simulink model "NO3_Multi_QuadcopterOffboard_Actuator"  (R2022a)
settings: Solver=FixedStepAuto  StartTime=0.0  StopTime=inf  RelTol=1e-3
undefined symbols (not defined in the file): actuator, command, control, param1, param2, target_system, timestamp
libraries: ros2lib x33
settings Model: Creator=liuwhale  LastModifiedBy=liuwhale
settings OptimizationCC: EnhancedBackFolding=on  PassReuseOutputArgsAs=Individual arguments  ZeroExternalMemoryAtStartup=off  ZeroInternalMemoryAtStartup=off  MaxStackSize=64  OptimizeBlockOrder=speed  DifferentSizesBufferReuse=on  OptimizationCustomize=off  EfficientTunableParamExpr=on
settings DebuggingCC: ParameterTunabilityLossMsg=error
settings SFSimCC: MATLABDynamicMemAlloc=off
settings RTWCC: SystemTargetFile=ert.tlc  HardwareBoard=Robot Operating System 2 (ROS 2)  TLCOptions="-aInlineSetEventsForThisBaseRateFcn=TLC_FALSE -aSuppressMultiTaskScheduler=TLC_FALSE  -aRateBasedStepFcn=0"  TemplateMakefile=ert_default_tmf  Toolchain=Colcon Tools  TargetLang=C++
settings CodeAppCC: ForceParamTrailComments=on  IgnoreCustomStorageClasses=off  OperatorAnnotations=on  SimulinkDataObjDesc=on  SFDataObjDesc=on  InsertBlockDesc=on
settings ERTTargetCC: CodeInterfacePackaging=C++ class  RootIOFormat=Structure reference

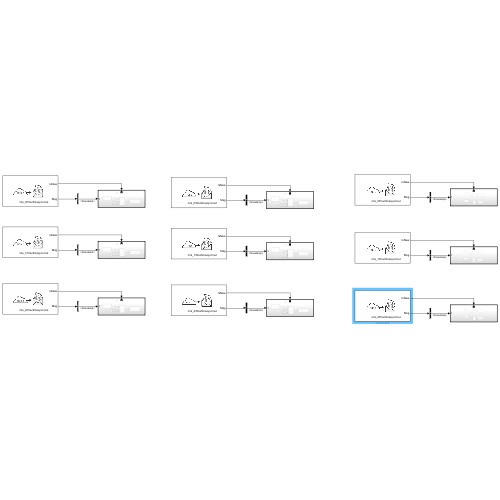
[thumbnail: Simulink's stored preview of the top-level diagram]
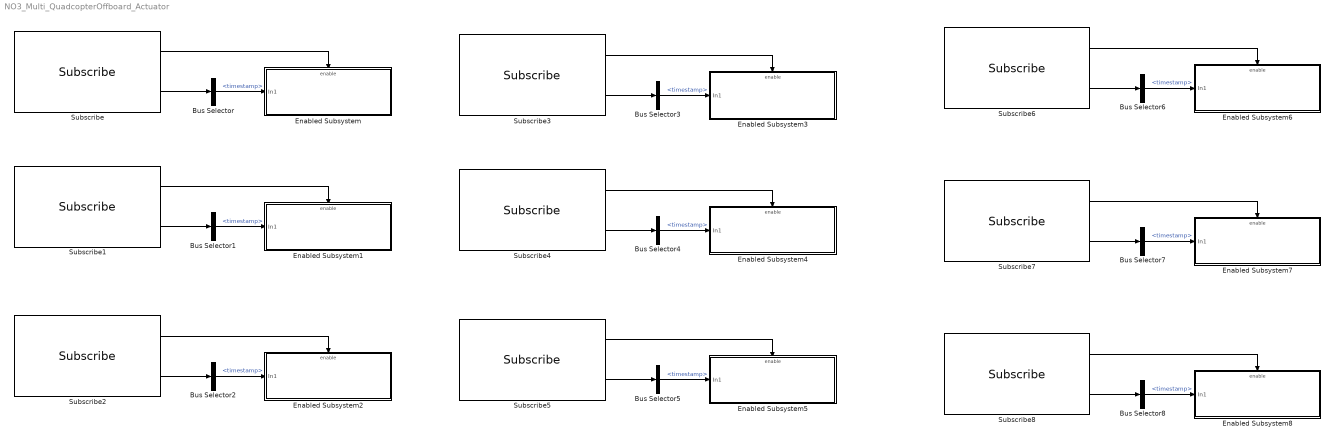
== system NO3_Multi_QuadcopterOffboard_Actuator ==
  Bus Selector{,1..8} (9 alike) : BusSelector  OutputSignals=timestamp
  Enabled Subsystem : Subsystem  TreatAsAtomicUnit=on
  Enabled Subsystem1 : Subsystem  TreatAsAtomicUnit=on
  Enabled Subsystem2 : Subsystem  TreatAsAtomicUnit=on
  Enabled Subsystem3 : Subsystem  TreatAsAtomicUnit=on
  Enabled Subsystem4 : Subsystem  TreatAsAtomicUnit=on
  Enabled Subsystem5 : Subsystem  TreatAsAtomicUnit=on
  Enabled Subsystem6 : Subsystem  TreatAsAtomicUnit=on
  Enabled Subsystem7 : Subsystem  TreatAsAtomicUnit=on
  Enabled Subsystem8 : Subsystem  TreatAsAtomicUnit=on
  Subscribe : ros2lib/Subscribe  topicSource=Specify your own  topic=/iris_0/fmu/timesync/out  messageType=px4_msgs/Timesync  sampleTime=-1  QOSHistory=Keep last  QOSDepth=1  QOSReliability=Reliable  QOSDurability=Volatile
      settings: SourceProductBaseCode=RR
  Subscribe1 : ros2lib/Subscribe  topicSource=Specify your own  topic=/iris_1/fmu/timesync/out  messageType=px4_msgs/Timesync  sampleTime=-1  QOSHistory=Keep last  QOSDepth=1  QOSReliability=Reliable  QOSDurability=Volatile
      settings: SourceProductBaseCode=RR
  Subscribe2 : ros2lib/Subscribe  topicSource=Specify your own  topic=/iris_2/fmu/timesync/out  messageType=px4_msgs/Timesync  sampleTime=-1  QOSHistory=Keep last  QOSDepth=1  QOSReliability=Reliable  QOSDurability=Volatile
      settings: SourceProductBaseCode=RR
  Subscribe3 : ros2lib/Subscribe  topicSource=Specify your own  topic=/iris_0/fmu/timesync/out  messageType=px4_msgs/Timesync  sampleTime=-1  QOSHistory=Keep last  QOSDepth=1  QOSReliability=Reliable  QOSDurability=Volatile
      settings: SourceProductBaseCode=RR
  Subscribe4 : ros2lib/Subscribe  topicSource=Specify your own  topic=/iris_1/fmu/timesync/out  messageType=px4_msgs/Timesync  sampleTime=-1  QOSHistory=Keep last  QOSDepth=1  QOSReliability=Reliable  QOSDurability=Volatile
      settings: SourceProductBaseCode=RR
  Subscribe5 : ros2lib/Subscribe  topicSource=Specify your own  topic=/iris_2/fmu/timesync/out  messageType=px4_msgs/Timesync  sampleTime=-1  QOSHistory=Keep last  QOSDepth=1  QOSReliability=Reliable  QOSDurability=Volatile
      settings: SourceProductBaseCode=RR
  Subscribe6 : ros2lib/Subscribe  topicSource=Specify your own  topic=/iris_0/fmu/timesync/out  messageType=px4_msgs/Timesync  sampleTime=-1  QOSHistory=Keep last  QOSDepth=1  QOSReliability=Reliable  QOSDurability=Volatile
      settings: SourceProductBaseCode=RR
  Subscribe7 : ros2lib/Subscribe  topicSource=Specify your own  topic=/iris_1/fmu/timesync/out  messageType=px4_msgs/Timesync  sampleTime=-1  QOSHistory=Keep last  QOSDepth=1  QOSReliability=Reliable  QOSDurability=Volatile
      settings: SourceProductBaseCode=RR
  Subscribe8 : ros2lib/Subscribe  topicSource=Specify your own  topic=/iris_2/fmu/timesync/out  messageType=px4_msgs/Timesync  sampleTime=-1  QOSHistory=Keep last  QOSDepth=1  QOSReliability=Reliable  QOSDurability=Volatile
      settings: SourceProductBaseCode=RR
  wires:
  Subscribe/1 -> Enabled Subsystem/Enable
  Subscribe/2 -> Bus Selector/1
  Bus Selector/1 -> Enabled Subsystem/1(In1)  "<timestamp>"
  Bus Selector1/1 -> Enabled Subsystem1/1(In1)  "<timestamp>"
  Subscribe1/2 -> Bus Selector1/1
  Subscribe1/1 -> Enabled Subsystem1/Enable
  Bus Selector2/1 -> Enabled Subsystem2/1(In1)  "<timestamp>"
  Subscribe2/2 -> Bus Selector2/1
  Subscribe2/1 -> Enabled Subsystem2/Enable
  Subscribe5/1 -> Enabled Subsystem5/Enable
  Bus Selector5/1 -> Enabled Subsystem5/1(In1)  "<timestamp>"
  Subscribe5/2 -> Bus Selector5/1
  Subscribe4/2 -> Bus Selector4/1
  Subscribe4/1 -> Enabled Subsystem4/Enable
  Bus Selector3/1 -> Enabled Subsystem3/1(In1)  "<timestamp>"
  Subscribe3/2 -> Bus Selector3/1
  Subscribe3/1 -> Enabled Subsystem3/Enable
  Bus Selector4/1 -> Enabled Subsystem4/1(In1)  "<timestamp>"
  Subscribe6/2 -> Bus Selector6/1
  Bus Selector6/1 -> Enabled Subsystem6/1(In1)  "<timestamp>"
  Subscribe6/1 -> Enabled Subsystem6/Enable
  Subscribe7/2 -> Bus Selector7/1
  Bus Selector7/1 -> Enabled Subsystem7/1(In1)  "<timestamp>"
  Subscribe8/2 -> Bus Selector8/1
  Bus Selector8/1 -> Enabled Subsystem8/1(In1)  "<timestamp>"
  Subscribe7/1 -> Enabled Subsystem7/Enable
  Subscribe8/1 -> Enabled Subsystem8/Enable

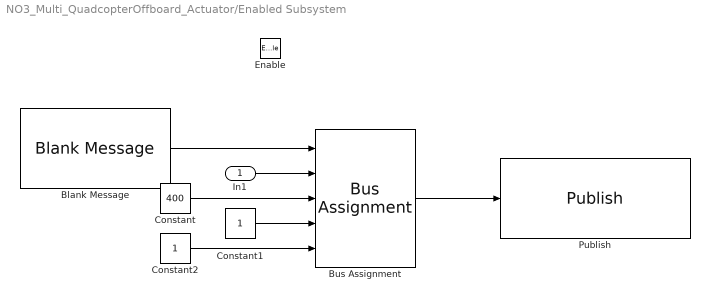
== system NO3_Multi_QuadcopterOffboard_Actuator/Enabled Subsystem ==
  In1 : Inport
  Enable : EnablePort
  Blank Message : ros2lib/Blank Message  messageClass=Message  entityType=px4_msgs/VehicleCommand  messageType=px4_msgs/VehicleCommand  SampleTime=inf
      settings: SourceProductBaseCode=RR
  Bus Assignment : BusAssignment  AssignedSignals=timestamp,command,param1,target_system
  Constant : Constant  Value=400  OutDataTypeStr=uint32
  Constant1 : Constant  OutDataTypeStr=single
  Constant2 : Constant  OutDataTypeStr=uint8
  Publish : ros2lib/Publish  topicSource=Specify your own  topic=/iris_0/fmu/vehicle_command/in  messageType=px4_msgs/VehicleCommand  QOSHistory=Keep last  QOSDepth=1  QOSReliability=Reliable  QOSDurability=Volatile
      settings: SourceProductBaseCode=RR
  wires:
  Blank Message/1 -> Bus Assignment/1
  In1/1 -> Bus Assignment/2
  Constant/1 -> Bus Assignment/3
  Constant1/1 -> Bus Assignment/4
  Constant2/1 -> Bus Assignment/5
  Bus Assignment/1 -> Publish/1

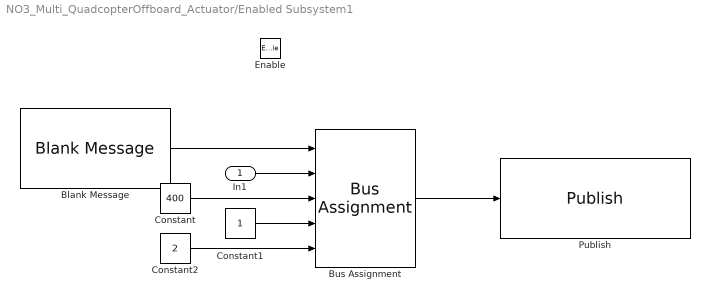
== system NO3_Multi_QuadcopterOffboard_Actuator/Enabled Subsystem1 ==
  In1 : Inport
  Enable : EnablePort
  Blank Message : ros2lib/Blank Message  messageClass=Message  entityType=px4_msgs/VehicleCommand  messageType=px4_msgs/VehicleCommand  SampleTime=inf
      settings: SourceProductBaseCode=RR
  Bus Assignment : BusAssignment  AssignedSignals=timestamp,command,param1,target_system
  Constant : Constant  Value=400  OutDataTypeStr=uint32
  Constant1 : Constant  OutDataTypeStr=single
  Constant2 : Constant  Value=2  OutDataTypeStr=uint8
  Publish : ros2lib/Publish  topicSource=Specify your own  topic=/iris_1/fmu/vehicle_command/in  messageType=px4_msgs/VehicleCommand  QOSHistory=Keep last  QOSDepth=1  QOSReliability=Reliable  QOSDurability=Volatile
      settings: SourceProductBaseCode=RR
  wires:
  Blank Message/1 -> Bus Assignment/1
  In1/1 -> Bus Assignment/2
  Constant/1 -> Bus Assignment/3
  Constant1/1 -> Bus Assignment/4
  Constant2/1 -> Bus Assignment/5
  Bus Assignment/1 -> Publish/1

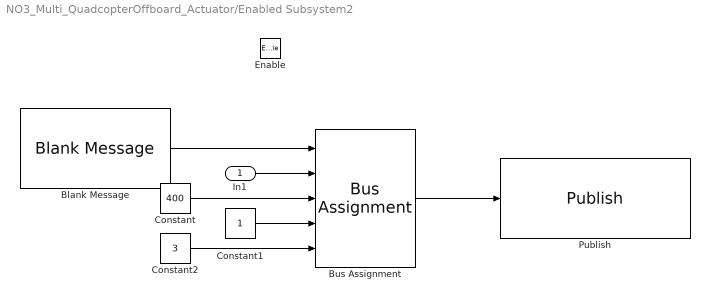
== system NO3_Multi_QuadcopterOffboard_Actuator/Enabled Subsystem2 ==
  In1 : Inport
  Enable : EnablePort
  Blank Message : ros2lib/Blank Message  messageClass=Message  entityType=px4_msgs/VehicleCommand  messageType=px4_msgs/VehicleCommand  SampleTime=inf
      settings: SourceProductBaseCode=RR
  Bus Assignment : BusAssignment  AssignedSignals=timestamp,command,param1,target_system
  Constant : Constant  Value=400  OutDataTypeStr=uint32
  Constant1 : Constant  OutDataTypeStr=single
  Constant2 : Constant  Value=3  OutDataTypeStr=uint8
  Publish : ros2lib/Publish  topicSource=Specify your own  topic=/iris_2/fmu/vehicle_command/in  messageType=px4_msgs/VehicleCommand  QOSHistory=Keep last  QOSDepth=1  QOSReliability=Reliable  QOSDurability=Volatile
      settings: SourceProductBaseCode=RR
  wires:
  Blank Message/1 -> Bus Assignment/1
  In1/1 -> Bus Assignment/2
  Constant/1 -> Bus Assignment/3
  Constant1/1 -> Bus Assignment/4
  Constant2/1 -> Bus Assignment/5
  Bus Assignment/1 -> Publish/1

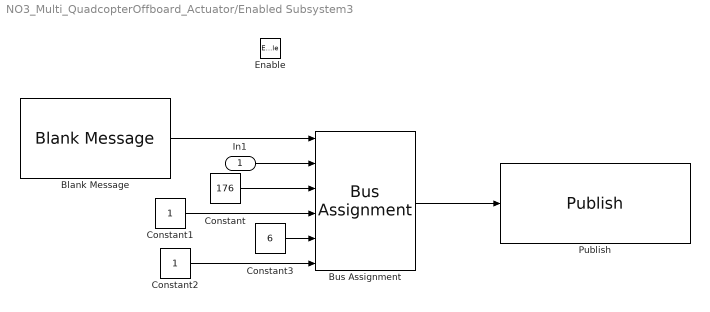
== system NO3_Multi_QuadcopterOffboard_Actuator/Enabled Subsystem3 ==
  In1 : Inport
  Enable : EnablePort
  Blank Message : ros2lib/Blank Message  messageClass=Message  entityType=px4_msgs/VehicleCommand  messageType=px4_msgs/VehicleCommand  SampleTime=inf
      settings: SourceProductBaseCode=RR
  Bus Assignment : BusAssignment  AssignedSignals=timestamp,command,param1,param2,target_system
  Constant : Constant  Value=176  OutDataTypeStr=uint32
  Constant1 : Constant  OutDataTypeStr=single
  Constant2 : Constant  OutDataTypeStr=uint8
  Constant3 : Constant  Value=6  OutDataTypeStr=single
  Publish : ros2lib/Publish  topicSource=Specify your own  topic=/iris_0/fmu/vehicle_command/in  messageType=px4_msgs/VehicleCommand  QOSHistory=Keep last  QOSDepth=1  QOSReliability=Reliable  QOSDurability=Volatile
      settings: SourceProductBaseCode=RR
  wires:
  Blank Message/1 -> Bus Assignment/1
  In1/1 -> Bus Assignment/2
  Constant/1 -> Bus Assignment/3
  Constant1/1 -> Bus Assignment/4
  Constant2/1 -> Bus Assignment/6
  Bus Assignment/1 -> Publish/1
  Constant3/1 -> Bus Assignment/5

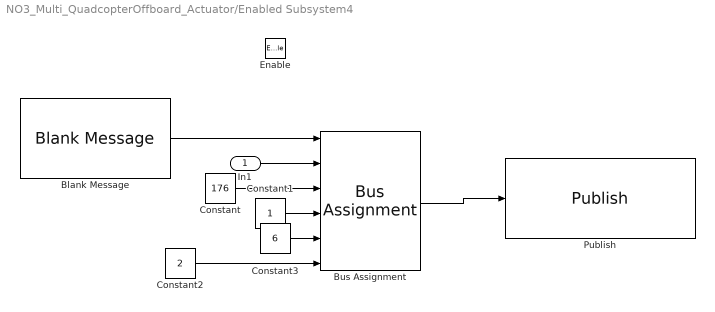
== system NO3_Multi_QuadcopterOffboard_Actuator/Enabled Subsystem4 ==
  In1 : Inport
  Enable : EnablePort
  Blank Message : ros2lib/Blank Message  messageClass=Message  entityType=px4_msgs/VehicleCommand  messageType=px4_msgs/VehicleCommand  SampleTime=inf
      settings: SourceProductBaseCode=RR
  Bus Assignment : BusAssignment  AssignedSignals=timestamp,command,param1,param2,target_system
  Constant : Constant  Value=176  OutDataTypeStr=uint32
  Constant1 : Constant  OutDataTypeStr=single
  Constant2 : Constant  Value=2  OutDataTypeStr=uint8
  Constant3 : Constant  Value=6  OutDataTypeStr=single
  Publish : ros2lib/Publish  topicSource=Specify your own  topic=/iris_1/fmu/vehicle_command/in  messageType=px4_msgs/VehicleCommand  QOSHistory=Keep last  QOSDepth=1  QOSReliability=Reliable  QOSDurability=Volatile
      settings: SourceProductBaseCode=RR
  wires:
  Blank Message/1 -> Bus Assignment/1
  In1/1 -> Bus Assignment/2
  Constant/1 -> Bus Assignment/3
  Constant1/1 -> Bus Assignment/4
  Constant2/1 -> Bus Assignment/6
  Bus Assignment/1 -> Publish/1
  Constant3/1 -> Bus Assignment/5

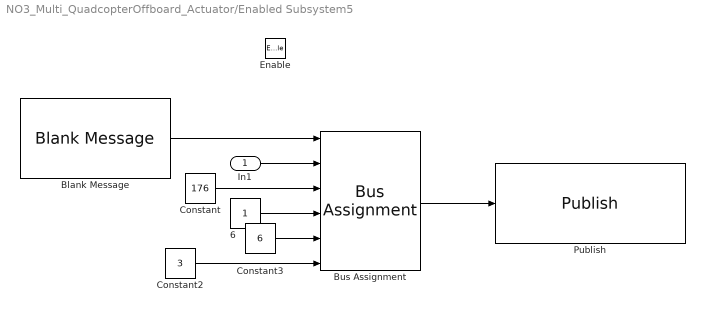
== system NO3_Multi_QuadcopterOffboard_Actuator/Enabled Subsystem5 ==
  In1 : Inport
  Enable : EnablePort
  6 : Constant  OutDataTypeStr=single
  Blank Message : ros2lib/Blank Message  messageClass=Message  entityType=px4_msgs/VehicleCommand  messageType=px4_msgs/VehicleCommand  SampleTime=inf
      settings: SourceProductBaseCode=RR
  Bus Assignment : BusAssignment  AssignedSignals=timestamp,command,param1,param2,target_system
  Constant : Constant  Value=176  OutDataTypeStr=uint32
  Constant2 : Constant  Value=3  OutDataTypeStr=uint8
  Constant3 : Constant  Value=6  OutDataTypeStr=single
  Publish : ros2lib/Publish  topicSource=Specify your own  topic=/iris_2/fmu/vehicle_command/in  messageType=px4_msgs/VehicleCommand  QOSHistory=Keep last  QOSDepth=1  QOSReliability=Reliable  QOSDurability=Volatile
      settings: SourceProductBaseCode=RR
  wires:
  Blank Message/1 -> Bus Assignment/1
  In1/1 -> Bus Assignment/2
  Constant/1 -> Bus Assignment/3
  6/1 -> Bus Assignment/4
  Constant2/1 -> Bus Assignment/6
  Bus Assignment/1 -> Publish/1
  Constant3/1 -> Bus Assignment/5

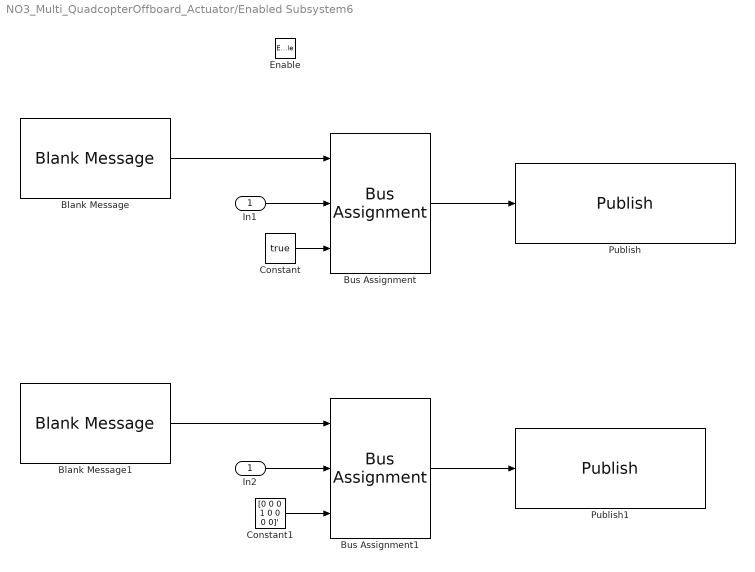
== system NO3_Multi_QuadcopterOffboard_Actuator/Enabled Subsystem6 ==
  In1 : Inport
  Enable : EnablePort
  Blank Message : ros2lib/Blank Message  messageClass=Message  entityType=px4_msgs/OffboardControlMode  messageType=px4_msgs/OffboardControlMode  SampleTime=inf
      settings: SourceProductBaseCode=RR
  Blank Message1 : ros2lib/Blank Message  messageClass=Message  entityType=px4_msgs/ActuatorControls0  messageType=px4_msgs/TrajectorySetpoint  SampleTime=inf
      settings: SourceProductBaseCode=RR
  Bus Assignment : BusAssignment  AssignedSignals=timestamp,actuator
  Bus Assignment1 : BusAssignment  AssignedSignals=timestamp,control
  Constant : Constant  Value=true  OutDataTypeStr=boolean
  Constant1 : Constant  Value=[0 0 0 1 0 0 0 0]'  OutDataTypeStr=single
  In2 : InportShadow
  Publish : ros2lib/Publish  topicSource=Specify your own  topic=/iris_0/fmu/offboard_control_mode/in  messageType=px4_msgs/OffboardControlMode  QOSHistory=Keep last  QOSDepth=1  QOSReliability=Reliable  QOSDurability=Volatile
      settings: SourceProductBaseCode=RR
  Publish1 : ros2lib/Publish  topicSource=Specify your own  topic=/iris_0/fmu/actuator_controls0/in  messageType=px4_msgs/ActuatorControls0  QOSHistory=Keep last  QOSDepth=1  QOSReliability=Reliable  QOSDurability=Volatile
      settings: SourceProductBaseCode=RR
  wires:
  Blank Message/1 -> Bus Assignment/1
  In1/1 -> Bus Assignment/2
  Bus Assignment/1 -> Publish/1
  Constant/1 -> Bus Assignment/3
  In2/1 -> Bus Assignment1/2
  Bus Assignment1/1 -> Publish1/1
  Blank Message1/1 -> Bus Assignment1/1
  Constant1/1 -> Bus Assignment1/3

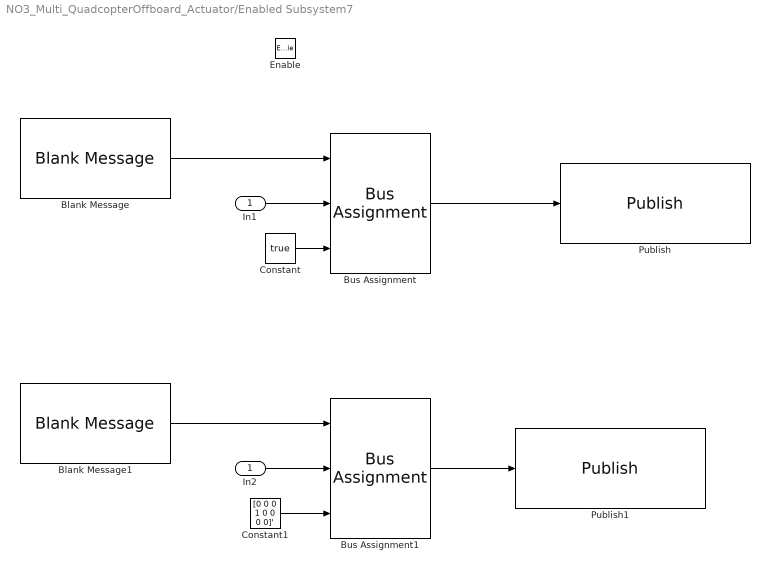
== system NO3_Multi_QuadcopterOffboard_Actuator/Enabled Subsystem7 ==
  In1 : Inport
  Enable : EnablePort
  Blank Message : ros2lib/Blank Message  messageClass=Message  entityType=px4_msgs/OffboardControlMode  messageType=px4_msgs/OffboardControlMode  SampleTime=inf
      settings: SourceProductBaseCode=RR
  Blank Message1 : ros2lib/Blank Message  messageClass=Message  entityType=px4_msgs/ActuatorControls0  messageType=px4_msgs/TrajectorySetpoint  SampleTime=inf
      settings: SourceProductBaseCode=RR
  Bus Assignment : BusAssignment  AssignedSignals=timestamp,actuator
  Bus Assignment1 : BusAssignment  AssignedSignals=timestamp,control
  Constant : Constant  Value=true  OutDataTypeStr=boolean
  Constant1 : Constant  Value=[0 0 0 1 0 0 0 0]'  OutDataTypeStr=single
  In2 : InportShadow
  Publish : ros2lib/Publish  topicSource=Specify your own  topic=/iris_1/fmu/offboard_control_mode/in  messageType=px4_msgs/OffboardControlMode  QOSHistory=Keep last  QOSDepth=1  QOSReliability=Reliable  QOSDurability=Volatile
      settings: SourceProductBaseCode=RR
  Publish1 : ros2lib/Publish  topicSource=Specify your own  topic=/iris_1/fmu/actuator_controls0/in  messageType=px4_msgs/ActuatorControls0  QOSHistory=Keep last  QOSDepth=1  QOSReliability=Reliable  QOSDurability=Volatile
      settings: SourceProductBaseCode=RR
  wires:
  Blank Message/1 -> Bus Assignment/1
  In1/1 -> Bus Assignment/2
  Bus Assignment/1 -> Publish/1
  Constant/1 -> Bus Assignment/3
  In2/1 -> Bus Assignment1/2
  Bus Assignment1/1 -> Publish1/1
  Blank Message1/1 -> Bus Assignment1/1
  Constant1/1 -> Bus Assignment1/3

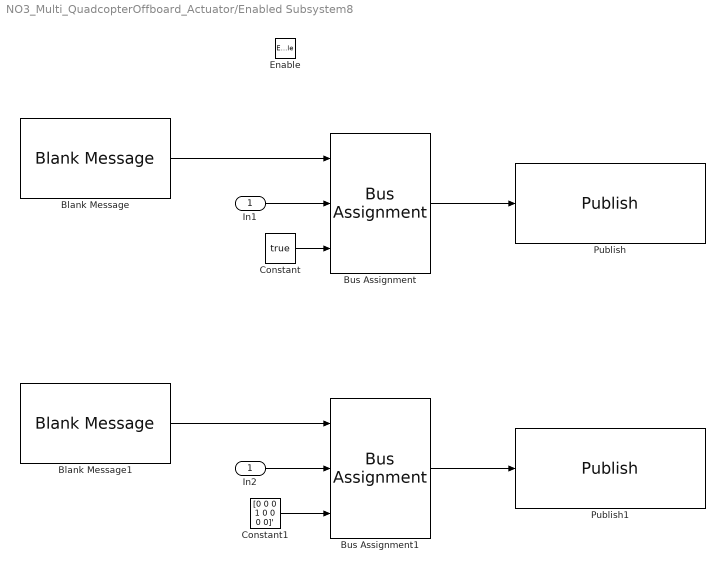
== system NO3_Multi_QuadcopterOffboard_Actuator/Enabled Subsystem8 ==
  In1 : Inport
  Enable : EnablePort
  Blank Message : ros2lib/Blank Message  messageClass=Message  entityType=px4_msgs/OffboardControlMode  messageType=px4_msgs/OffboardControlMode  SampleTime=inf
      settings: SourceProductBaseCode=RR
  Blank Message1 : ros2lib/Blank Message  messageClass=Message  entityType=px4_msgs/ActuatorControls0  messageType=px4_msgs/TrajectorySetpoint  SampleTime=inf
      settings: SourceProductBaseCode=RR
  Bus Assignment : BusAssignment  AssignedSignals=timestamp,actuator
  Bus Assignment1 : BusAssignment  AssignedSignals=timestamp,control
  Constant : Constant  Value=true  OutDataTypeStr=boolean
  Constant1 : Constant  Value=[0 0 0 1 0 0 0 0]'  OutDataTypeStr=single
  In2 : InportShadow
  Publish : ros2lib/Publish  topicSource=Specify your own  topic=/iris_2/fmu/offboard_control_mode/in  messageType=px4_msgs/OffboardControlMode  QOSHistory=Keep last  QOSDepth=1  QOSReliability=Reliable  QOSDurability=Volatile
      settings: SourceProductBaseCode=RR
  Publish1 : ros2lib/Publish  topicSource=Specify your own  topic=/iris_2/fmu/actuator_controls0/in  messageType=px4_msgs/ActuatorControls0  QOSHistory=Keep last  QOSDepth=1  QOSReliability=Reliable  QOSDurability=Volatile
      settings: SourceProductBaseCode=RR
  wires:
  Blank Message/1 -> Bus Assignment/1
  In1/1 -> Bus Assignment/2
  Bus Assignment/1 -> Publish/1
  Constant/1 -> Bus Assignment/3
  In2/1 -> Bus Assignment1/2
  Bus Assignment1/1 -> Publish1/1
  Blank Message1/1 -> Bus Assignment1/1
  Constant1/1 -> Bus Assignment1/3
